simulink model "tarea3"  (R2017b)
settings: Solver=VariableStepAuto  StartTime=0.0  StopTime=10.0  RelTol=1e-3
settings Model: Creator=Fanny  LastModifiedBy=Fanny

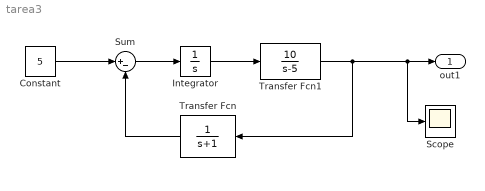
== system tarea3 ==
  Constant : Constant  Value=5
  Integrator : Integrator
  Scope : Scope
  Sum : Sum  Inputs=|+-
  Transfer Fcn : TransferFcn  Denominator=[1 1]
  Transfer Fcn1 : TransferFcn  Numerator=[10]  Denominator=[1 -5]
  "out1 " : Outport
  wires:
  Sum/1 -> Integrator/1
  Integrator/1 -> Transfer Fcn1/1
  Transfer Fcn1/1 -> Scope/1, "out1 "/1, Transfer Fcn/1
  Transfer Fcn/1 -> Sum/2
  Constant/1 -> Sum/1
